simulink model "sscv_braking_ABS_w_vehicle"  (R2024a)
settings: Solver=ode23t  StartTime=0.0  StopTime=1  RelTol=1e-3  AbsTol=1e-3
PreLoadFcn:
  | sscv_braking_ABS_w_vehicle_input
values from neighbouring files (symbols this model uses):
  wheel_rad = 0.3    [sscv_braking_ABS_w_vehicle_input.m]
  wheel_vth = 0.01    [sscv_braking_ABS_w_vehicle_input.m]
undefined symbols (not defined in the file or in its folder): Asphalt, fcdb, HCU, MFormulaCoeff, tpc, vb
libraries: fl_lib x165, SimscapeFluids_lib x24, nesl_utility x21, sdl_lib x9, simulink x3, simulink_extras x1
(part 4 of 6)

== system sscv_braking_ABS_w_vehicle/Road Surface/Road/Select MF Coefficients ==
  Surface : Inport
  Dry Tarmac : Constant  Value=MFormulaCoeff.DryTarmac  SampleTime=0
  Filter MF Coeff LF : Subsystem  mask(First-order lag supporting vector signals){b=0.01, x_initial=MFormulaCoeff.DryTarmac}
      mask prompts: b "Filter time constant"; x_initial "Initial output"
      mask help: Models a lag of the form 1/(b*s+1) where s is the Laplace operator.
  Filter MF Coeff LR : Subsystem  mask(First-order lag supporting vector signals){b=0.01, x_initial=MFormulaCoeff.DryTarmac}
      mask prompts: b "Filter time constant"; x_initial "Initial output"
      mask help: Models a lag of the form 1/(b*s+1) where s is the Laplace operator.
  Filter MF Coeff RF : Subsystem  mask(First-order lag supporting vector signals){b=0.01, x_initial=MFormulaCoeff.DryTarmac}
      mask prompts: b "Filter time constant"; x_initial "Initial output"
      mask help: Models a lag of the form 1/(b*s+1) where s is the Laplace operator.
  Filter MF Coeff RR : Subsystem  mask(First-order lag supporting vector signals){b=0.01, x_initial=MFormulaCoeff.DryTarmac}
      mask prompts: b "Filter time constant"; x_initial "Initial output"
      mask help: Models a lag of the form 1/(b*s+1) where s is the Laplace operator.
  Ice : Constant  Value=MFormulaCoeff.Ice  SampleTime=0
  Select Coeff : Subsystem
  Snow : Constant  Value=MFormulaCoeff.Snow  SampleTime=0
  Wet Tarmac : Constant  Value=MFormulaCoeff.WetTarmac  SampleTime=0
  LF : Outport  VectorParamsAs1DForOutWhenUnconnected=off
  RF : Outport  Port=2  VectorParamsAs1DForOutWhenUnconnected=off
  LR : Outport  Port=3  VectorParamsAs1DForOutWhenUnconnected=off
  RR : Outport  Port=4  VectorParamsAs1DForOutWhenUnconnected=off
  wires:
  Select Coeff/2(RF) -> Filter MF Coeff RF/1(In)
  Select Coeff/1(LF) -> Filter MF Coeff LF/1(In)
  Select Coeff/4(RR) -> Filter MF Coeff RR/1(In)
  Select Coeff/3(LR) -> Filter MF Coeff LR/1(In)
  Surface/1 -> Select Coeff/1(Surface)
  Snow/1 -> Select Coeff/3(Snow)
  Wet Tarmac/1 -> Select Coeff/4(Wet)
  Ice/1 -> Select Coeff/2(Ice)
  Dry Tarmac/1 -> Select Coeff/5(Dry)
  Filter MF Coeff LF/1(Out) -> LF/1
  Filter MF Coeff RF/1(Out) -> RF/1
  Filter MF Coeff LR/1(Out) -> LR/1
  Filter MF Coeff RR/1(Out) -> RR/1

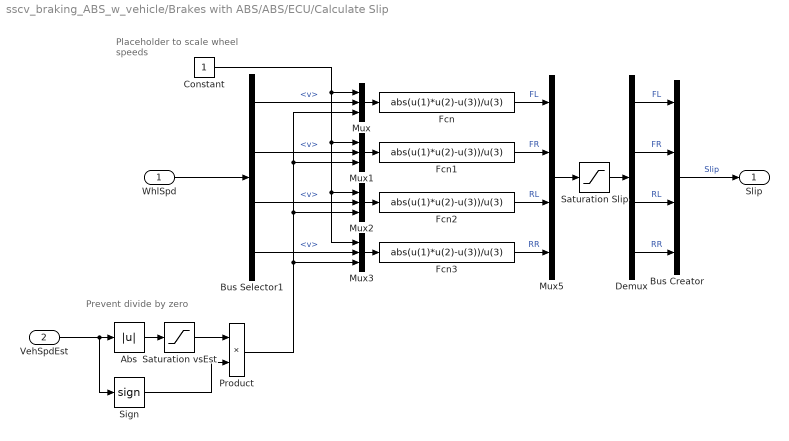
== system sscv_braking_ABS_w_vehicle/Brakes with ABS/ABS/ECU/Calculate Slip ==
  note: Placeholder
      | to scale
      | wheel speeds
  note: Prevent divide by zero
  WhlSpd : Inport
  VehSpdEst : Inport  Port=2
  Abs : Abs  ZeroCross=off  SaturateOnIntegerOverflow=off
  Bus Creator : BusCreator  Inputs=4
  Bus Selector1 : BusSelector  OutputSignals=FL.v,FR.v,RL.v,RR.v
  Constant : Constant
  Demux : Demux
  Fcn{,1..3} (4 alike) : Fcn  Expr=abs(u(1)*u(2)-u(3))/u(3)
  Mux{,1..3} (4 alike) : Mux  Inputs=3
  Mux5 : Mux
  Product : Product
  Saturation Slip : Saturate  UpperLimit=1  LowerLimit=0
  Saturation vsEst : Saturate  UpperLimit=inf  LowerLimit=eps  ZeroCross=off
  Sign : Signum  ZeroCross=off
  Slip : Outport  VectorParamsAs1DForOutWhenUnconnected=off
  wires:
  WhlSpd/1 -> Bus Selector1/1
  Bus Selector1/2 -> Mux1/2  "<v>"
  Bus Selector1/4 -> Mux3/2  "<v>"
  Bus Selector1/1 -> Mux/2  "<v>"
  Bus Selector1/3 -> Mux2/2  "<v>"
  Constant/1 -> Mux1/1, Mux3/1, Mux2/1, Mux/1
  VehSpdEst/1 -> Sign/1, Abs/1
  Demux/1 -> Bus Creator/1  "FL"
  Demux/2 -> Bus Creator/2  "FR"
  Demux/3 -> Bus Creator/3  "RL"
  Demux/4 -> Bus Creator/4  "RR"
  Bus Creator/1 -> Slip/1  "Slip"
  Product/1 -> Mux3/3, Mux2/3, Mux1/3, Mux/3
  Abs/1 -> Saturation vsEst/1
  Saturation vsEst/1 -> Product/1
  Sign/1 -> Product/2
  Mux/1 -> Fcn/1
  Mux1/1 -> Fcn1/1
  Mux2/1 -> Fcn2/1
  Mux3/1 -> Fcn3/1
  Mux5/1 -> Saturation Slip/1
  Saturation Slip/1 -> Demux/1
  Fcn/1 -> Mux5/1  "FL"
  Fcn1/1 -> Mux5/2  "FR"
  Fcn2/1 -> Mux5/3  "RL"
  Fcn3/1 -> Mux5/4  "RR"

== system sscv_braking_ABS_w_vehicle/Brakes with ABS/ABS/ECU/Valve Control FL ==
  Slip : Inport
  vSpdEst : Inport  Port=2
  Code to Valves : Subsystem
  Demux : Demux  Outputs=2
  Logic : Stateflow chart  TreatAsAtomicUnit=on
  Mux : Mux  Inputs=2
  Product : Product
  Subsystem : Subsystem
  Subsystem1 : Subsystem
  Valve : Outport  VectorParamsAs1DForOutWhenUnconnected=off
  wires:
  Subsystem1/1(vSig) -> Mux/2
  Subsystem/1(vSig) -> Mux/1
  Mux/1 -> Valve/1
  Demux/2 -> Subsystem1/1(OnT)
  Demux/1 -> Subsystem/1(OnT)
  Product/1 -> Demux/1
  vSpdEst/1 -> Logic/2(vSpdEst)
  Code to Valves/1(V) -> Product/1
  Slip/1 -> Logic/1(Slip)
  Logic/2(Mod_Dur) -> Product/2
  Logic/1(Mod_State) -> Code to Valves/1(C)

== system sscv_braking_ABS_w_vehicle/Brakes with ABS/ABS/ECU/Valve Control FR ==
  Slip : Inport
  vSpdEst : Inport  Port=2
  Code to Valves : Subsystem
  Demux : Demux  Outputs=2
  Logic : Stateflow chart  TreatAsAtomicUnit=on
  Mux : Mux  Inputs=2
  Product : Product
  Subsystem : Subsystem
  Subsystem1 : Subsystem
  Valve : Outport  VectorParamsAs1DForOutWhenUnconnected=off
  wires:
  Subsystem1/1(vSig) -> Mux/2
  Subsystem/1(vSig) -> Mux/1
  Mux/1 -> Valve/1
  Demux/2 -> Subsystem1/1(OnT)
  Demux/1 -> Subsystem/1(OnT)
  Product/1 -> Demux/1
  vSpdEst/1 -> Logic/2(vSpdEst)
  Code to Valves/1(V) -> Product/1
  Slip/1 -> Logic/1(Slip)
  Logic/2(Mod_Dur) -> Product/2
  Logic/1(Mod_State) -> Code to Valves/1(C)

== system sscv_braking_ABS_w_vehicle/Brakes with ABS/ABS/ECU/Valve Control RL ==
  Slip : Inport
  vSpdEst : Inport  Port=2
  Code to Valves : Subsystem
  Demux : Demux  Outputs=2
  Logic : Stateflow chart  TreatAsAtomicUnit=on
  Mux : Mux  Inputs=2
  Product : Product
  Subsystem : Subsystem
  Subsystem1 : Subsystem
  Valve : Outport  VectorParamsAs1DForOutWhenUnconnected=off
  wires:
  Subsystem1/1(vSig) -> Mux/2
  Subsystem/1(vSig) -> Mux/1
  Mux/1 -> Valve/1
  Demux/2 -> Subsystem1/1(OnT)
  Demux/1 -> Subsystem/1(OnT)
  Product/1 -> Demux/1
  vSpdEst/1 -> Logic/2(vSpdEst)
  Code to Valves/1(V) -> Product/1
  Slip/1 -> Logic/1(Slip)
  Logic/2(Mod_Dur) -> Product/2
  Logic/1(Mod_State) -> Code to Valves/1(C)

== system sscv_braking_ABS_w_vehicle/Brakes with ABS/ABS/ECU/Valve Control RR ==
  Slip : Inport
  vSpdEst : Inport  Port=2
  Code to Valves : Subsystem
  Demux : Demux  Outputs=2
  Logic : Stateflow chart  TreatAsAtomicUnit=on
  Mux : Mux  Inputs=2
  Product : Product
  Subsystem : Subsystem
  Subsystem1 : Subsystem
  Valve : Outport  VectorParamsAs1DForOutWhenUnconnected=off
  wires:
  Subsystem1/1(vSig) -> Mux/2
  Subsystem/1(vSig) -> Mux/1
  Mux/1 -> Valve/1
  Demux/2 -> Subsystem1/1(OnT)
  Demux/1 -> Subsystem/1(OnT)
  Product/1 -> Demux/1
  vSpdEst/1 -> Logic/2(vSpdEst)
  Code to Valves/1(V) -> Product/1
  Slip/1 -> Logic/1(Slip)
  Logic/2(Mod_Dur) -> Product/2
  Logic/1(Mod_State) -> Code to Valves/1(C)

== system sscv_braking_ABS_w_vehicle/Brakes with ABS/ABS/ECU/Vehicle Speed ==
  note: Estimates wheel speed using only wheel speed sensors and longitudinal accelerometer.
  note: Longitudinal
      | Accelerometer
  Sensors : Inport
  Accelerometer : simulink_extras/Additional Linear/Transfer Fcn (with initial states)  N=[1 0]  D="[0.01  1]"  X0=0
  Bus Selector : BusSelector  OutputSignals=v
  Bus Selector1 : BusSelector  OutputSignals=FL.v,FR.v,RL.v,RR.v
  Dynamic Rate Limiter : Subsystem
  Max : MinMax  Function=max  Inputs=4
  Rate Limit high : Constant  Value=8
  Saturation : Saturate  UpperLimit=0  LowerLimit=-inf
  ZOH rate limit low : ZeroOrderHold  SampleTime=1e-2
  ZOH vel : ZeroOrderHold  SampleTime=1e-2
  vSpdEst : Outport  VectorParamsAs1DForOutWhenUnconnected=off
  wires:
  Sensors/1 -> Bus Selector/1, Bus Selector1/1
  Bus Selector/1 -> Accelerometer/1  "<v>"
  Bus Selector1/1 -> Max/1  "<v>"
  Bus Selector1/2 -> Max/2  "<v>"
  Bus Selector1/3 -> Max/3  "<v>"
  Bus Selector1/4 -> Max/4  "<v>"
  Max/1 -> ZOH vel/1  "Max Wheel Spd"
  ZOH vel/1 -> Dynamic Rate Limiter/2(u)
  ZOH rate limit low/1 -> Dynamic Rate Limiter/3(lo)
  Rate Limit high/1 -> Dynamic Rate Limiter/1(up)
  Dynamic Rate Limiter/1(Y) -> vSpdEst/1  "vSpdEst"
  Accelerometer/1 -> Saturation/1
  Saturation/1 -> ZOH rate limit low/1

== system sscv_braking_ABS_w_vehicle/Brakes with ABS/ABS/HCU/Actuator Dynamics FL ==
  In : Inport
  Gain : Gain  Gain=1./b
  Integrator : Integrator  InitialCondition=x_initial.*b
  Sum : Sum  Inputs=|+-  InputSameDT=on  SaturateOnIntegerOverflow=on  OutDataTypeStr=Inherit: Same as first input
  Out : Outport  VectorParamsAs1DForOutWhenUnconnected=off
  wires:
  Sum/1 -> Integrator/1
  In/1 -> Sum/1
  Integrator/1 -> Gain/1
  Gain/1 -> Sum/2, Out/1

== system sscv_braking_ABS_w_vehicle/Brakes with ABS/ABS/HCU/Actuator Dynamics FR ==
  In : Inport
  Gain : Gain  Gain=1./b
  Integrator : Integrator  InitialCondition=x_initial.*b
  Sum : Sum  Inputs=|+-  InputSameDT=on  SaturateOnIntegerOverflow=on  OutDataTypeStr=Inherit: Same as first input
  Out : Outport  VectorParamsAs1DForOutWhenUnconnected=off
  wires:
  Gain/1 -> Out/1, Sum/2
  Integrator/1 -> Gain/1
  In/1 -> Sum/1
  Sum/1 -> Integrator/1

== system sscv_braking_ABS_w_vehicle/Brakes with ABS/ABS/HCU/Actuator Dynamics RL ==
  In : Inport
  Gain : Gain  Gain=1./b
  Integrator : Integrator  InitialCondition=x_initial.*b
  Sum : Sum  Inputs=|+-  InputSameDT=on  SaturateOnIntegerOverflow=on  OutDataTypeStr=Inherit: Same as first input
  Out : Outport  VectorParamsAs1DForOutWhenUnconnected=off
  wires:
  Gain/1 -> Out/1, Sum/2
  Integrator/1 -> Gain/1
  In/1 -> Sum/1
  Sum/1 -> Integrator/1

== system sscv_braking_ABS_w_vehicle/Brakes with ABS/ABS/HCU/Actuator Dynamics RR ==
  In : Inport
  Gain : Gain  Gain=1./b
  Integrator : Integrator  InitialCondition=x_initial.*b
  Sum : Sum  Inputs=|+-  InputSameDT=on  SaturateOnIntegerOverflow=on  OutDataTypeStr=Inherit: Same as first input
  Out : Outport  VectorParamsAs1DForOutWhenUnconnected=off
  wires:
  Gain/1 -> Out/1, Sum/2
  Integrator/1 -> Gain/1
  In/1 -> Sum/1
  Sum/1 -> Integrator/1

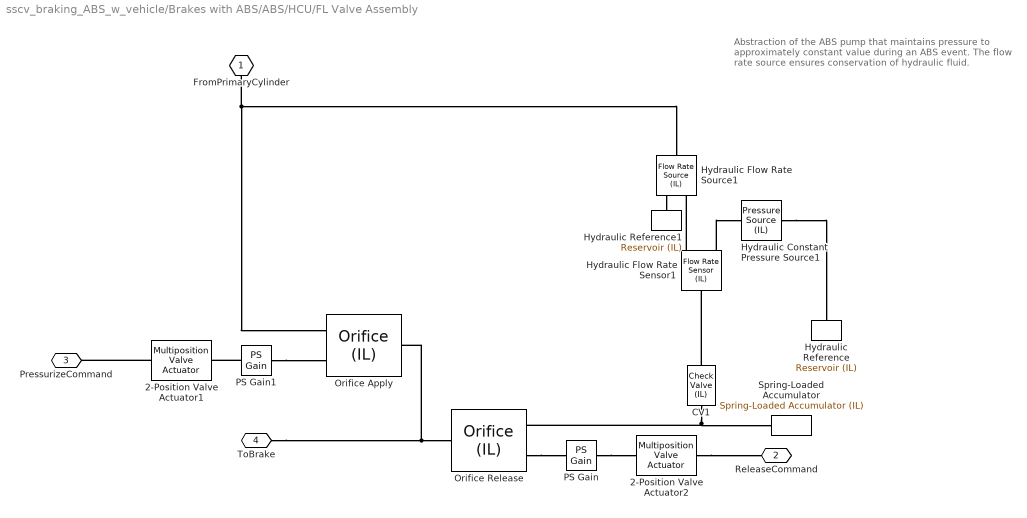
== system sscv_braking_ABS_w_vehicle/Brakes with ABS/ABS/HCU/FL Valve Assembly ==
  note: Abstraction of the ABS pump
      | that maintains pressure to
      | approximately constant value
      | during an ABS event. The
      | flow rate source ensures
      | conservation of hydraulic fluid.
  2-Position Valve Actuator1 : SimscapeFluids_lib/Valve Actuators/Multiposition Valve Actuator  positions=fluids.valve_actuators.enum.actuator_num_positions.two  stroke=HCU.PushPinS m  t_on=HCU.SwitchOnT s  t_off=HCU.SwitchOffT s  act_signal=HCU.NomSigV  init_position_2=0  init_position_3=fluids.valve_actuators.enum.actuator_three_pos_ic.neutral  act_orientation=1  local_time_specify=off  local_time_priority=None  local_time=0 s  local_time_nominal_specify=off  local_time_nominal_value=1  local_time_nominal_unit=s
      settings: InternalSimscapePortConfiguration="{\"Bottom\":[],\"Left\":[{\"id\":\"A\",\"label\":\"A\",\"type\":\"input\"}],\"Right\":[{\"id\":\"S\",\"label\":\"S\",\"type\":\"output\"}],\"Top\":[]}"
  2-Position Valve Actuator2 : SimscapeFluids_lib/Valve Actuators/Multiposition Valve Actuator  positions=fluids.valve_actuators.enum.actuator_num_positions.two  stroke=HCU.PushPinS m  t_on=HCU.SwitchOnT s  t_off=HCU.SwitchOffT s  act_signal=HCU.NomSigV  init_position_2=0  init_position_3=fluids.valve_actuators.enum.actuator_three_pos_ic.neutral  act_orientation=1  local_time_specify=off  local_time_priority=None  local_time=0 s  local_time_nominal_specify=off  local_time_nominal_value=1  local_time_nominal_unit=s
      settings: InternalSimscapePortConfiguration="{\"Bottom\":[],\"Left\":[{\"id\":\"A\",\"label\":\"A\",\"type\":\"input\"}],\"Right\":[{\"id\":\"S\",\"label\":\"S\",\"type\":\"output\"}],\"Top\":[]}"
  CV1 : SimscapeFluids_lib/Isothermal Liquid/Valves & Orifices/Directional Control Valves/Check Valve (IL)  opening_spec=fluids.isothermal_liquid.valves_orifices.enum.PressureOpeningSpec.Linear  pressure_control_spec=fluids.isothermal_liquid.valves_orifices.enum.pressure_control_spec.dp  p_crack_differential=HCU.cv1CrackP Pa  p_crack_gauge=0.1 MPa  press_max_differential=HCU.cv1MaxOpP Pa  press_max_gauge=0.2 MPa  area_max=HCU.cv1Amax m^2  area_leak=1e-8 m^2  p_diff_TLU=[0.01 : 0.01 : 0.1] MPa  valve_area_TLU=[1e-10, 1e-05, 2e-05, 3e-05, 4e-05, 5e-05, 6e-05, 7.5e-05, 8.5e-05, .0001] m^2  vol_flow_TLU=[.000358, .045, .11, .191, .284, .39, .505, .63, .764, .905] .* 1e-3 m^3/s  area=inf m^2  Cd=0.7  Re_c=150  smoothing_factor=0  pressure_recovery=simscape.enum.onoff.off  opening_dynamics=0  tau=0.1 s  enable_faults=simscape.enum.onoff.off  fault_action=fluids.enum.FaultOpening.Closed
      settings: InternalSimscapePortConfiguration="{\"Bottom\":[],\"Left\":[{\"id\":\"A\",\"label\":\"A\",\"type\":\"foundation.isothermal_liquid.isothermal_liquid\"}],\"Right\":[{\"id\":\"B\",\"label\":\"B\",\"type\":\"foundation.isothermal_liquid.isothermal_liquid\"}],\"Top\":[]}"
  Hydraulic Constant Pressure Source1 : fl_lib/Isothermal Liquid/Sources/Pressure Source (IL)  source_type=1  pressure_differential=1 atm
      settings: InternalSimscapePortConfiguration="{\"Bottom\":[],\"Left\":[{\"id\":\"A\",\"label\":\"A\",\"type\":\"foundation.isothermal_liquid.isothermal_liquid\"}],\"Right\":[{\"id\":\"B\",\"label\":\"B\",\"type\":\"foundation.isothermal_liquid.isothermal_liquid\"}],\"Top\":[]}"
  Hydraulic Flow Rate Sensor1 : fl_lib/Isothermal Liquid/Sensors/Flow Rate Sensor (IL)  sensor_type=3
      settings: InternalSimscapePortConfiguration="{\"Bottom\":[],\"Left\":[{\"id\":\"A\",\"label\":\"A\",\"type\":\"foundation.isothermal_liquid.isothermal_liquid\"}],\"Right\":[{\"id\":\"B\",\"label\":\"B\",\"type\":\"foundation.isothermal_liquid.isothermal_liquid\"},{\"id\":\"M\",\"label\":\"M\",\"type\":\"output\"},{\"id\":\"V\",\"label\":\"V\",\"type\":\"output\"}],\"Top\":[]}"
  Hydraulic Flow Rate Source1 : fl_lib/Isothermal Liquid/Sources/Flow Rate Source (IL)  source_type=foundation.enum.constant_controlled.controlled  flow_type=2  mass_flow=0 kg/s  volumetric_flow=0 m^3/s
      settings: InternalSimscapePortConfiguration="{\"Bottom\":[],\"Left\":[{\"id\":\"A\",\"label\":\"A\",\"type\":\"foundation.isothermal_liquid.isothermal_liquid\"},{\"id\":\"V\",\"label\":\"V\",\"type\":\"input\"}],\"Right\":[{\"id\":\"B\",\"label\":\"B\",\"type\":\"foundation.isothermal_liquid.isothermal_liquid\"}],\"Top\":[]}"
  Hydraulic Reference : fl_lib/Isothermal Liquid/Elements/Reservoir (IL)  reservoir_type=foundation.enum.constant_controlled.constant  pressure_spec=foundation.enum.pressure_spec.atmospheric  reservoir_pressure=0.101325 MPa
  Hydraulic Reference1 : fl_lib/Isothermal Liquid/Elements/Reservoir (IL)  reservoir_type=foundation.enum.constant_controlled.constant  pressure_spec=foundation.enum.pressure_spec.atmospheric  reservoir_pressure=0.101325 MPa
  Orifice Apply : SimscapeFluids_lib/Isothermal Liquid/Valves & Orifices/Orifices/Orifice (IL)  orifice_type=foundation.enum.constant_variable.variable  constant_orifice_spec=fluids.isothermal_liquid.valves_orifices.orifices.enum.constant_orifice_spec.area  variable_orifice_spec=1  orifice_area_constant=1e-3 m^2  p_diff_TLU_constant=[-4, -3, -2, -1, -.5, 0, .5, 1, 2, 3, 4] MPa  vol_flow_TLU_constant=[-2.44, -2.12, -1.68, -1.22, -.84, 0, .85, 1.21, 1.7, 2.09, 2.41] .* 1e-3 m^3/s  S_min=HCU.valve_x0 m  del_S=HCU.valve_maxO m  open_orientation=1  area_max=HCU.valve_maxA m^2  area_leak=HCU.valve_leak m^2  S_TLU=[-.002, 0, .002, .005, .015] - (HCU.valve_x0) m  orifice_area_TLU=[1e-09, 2.0352e-07, 4.0736e-05, .00011438, .00034356] m^2  area=inf m^2  Cd=0.7  Re_c=150  smoothing_factor=0  pressure_recovery=simscape.enum.onoff.off  S_vol_flow_TLU=[-.002, 0, .002, .005, .015] - (HCU.valve_x0) m  p_diff_TLU=[-10000000, -5000000, -2000000, 2000000, 5000000, 10000000] Pa  vol_flow_TLU=[-1e-07, -7.0711e-08, -4.4721e-08, 4.4721e-08, 7.0711e-08, 1e-07; -2.0352e-05, -1.4391e-05, -9.1017e-06, 9.1017e-06, 1.4391e-05, 2.0352e-05; -.0040736, -.0028805, -.0018218, .0018218, .0028805, .0040736; -.011438, -.0080879, -.0051152, .0051152, .0080879, .011438; -.034356, -.024293, -.015364, .015364, .024293, .034356] m^3/s  enable_faults=simscape.enum.onoff.off  fault_action=fluids.enum.FaultOpening.Closed
      settings: InternalSimscapePortConfiguration="{\"Bottom\":[],\"Left\":[{\"id\":\"A\",\"label\":\"A\",\"type\":\"foundation.isothermal_liquid.isothermal_liquid\"},{\"id\":\"S\",\"label\":\"S\",\"type\":\"input\"}],\"Right\":[{\"id\":\"B\",\"label\":\"B\",\"type\":\"foundation.isothermal_liquid.isothermal_liquid\"}],\"Top\":[]}"
  Orifice Release : SimscapeFluids_lib/Isothermal Liquid/Valves & Orifices/Orifices/Orifice (IL)  orifice_type=foundation.enum.constant_variable.variable  constant_orifice_spec=fluids.isothermal_liquid.valves_orifices.orifices.enum.constant_orifice_spec.area  variable_orifice_spec=1  orifice_area_constant=1e-3 m^2  p_diff_TLU_constant=[-4, -3, -2, -1, -.5, 0, .5, 1, 2, 3, 4] MPa  vol_flow_TLU_constant=[-2.44, -2.12, -1.68, -1.22, -.84, 0, .85, 1.21, 1.7, 2.09, 2.41] .* 1e-3 m^3/s  S_min=HCU.valve_x0 m  del_S=HCU.valve_maxO m  open_orientation=1  area_max=HCU.valve_maxA m^2  area_leak=HCU.valve_leak m^2  S_TLU=[-.002, 0, .002, .005, .015] - (HCU.valve_x0) m  orifice_area_TLU=[1e-09, 2.0352e-07, 4.0736e-05, .00011438, .00034356] m^2  area=inf m^2  Cd=0.7  Re_c=150  smoothing_factor=0  pressure_recovery=simscape.enum.onoff.off  S_vol_flow_TLU=[-.002, 0, .002, .005, .015] - (HCU.valve_x0) m  p_diff_TLU=[-10000000, -5000000, -2000000, 2000000, 5000000, 10000000] Pa  vol_flow_TLU=[-1e-07, -7.0711e-08, -4.4721e-08, 4.4721e-08, 7.0711e-08, 1e-07; -2.0352e-05, -1.4391e-05, -9.1017e-06, 9.1017e-06, 1.4391e-05, 2.0352e-05; -.0040736, -.0028805, -.0018218, .0018218, .0028805, .0040736; -.011438, -.0080879, -.0051152, .0051152, .0080879, .011438; -.034356, -.024293, -.015364, .015364, .024293, .034356] m^3/s  enable_faults=simscape.enum.onoff.off  fault_action=fluids.enum.FaultOpening.Closed
      settings: InternalSimscapePortConfiguration="{\"Bottom\":[],\"Left\":[{\"id\":\"A\",\"label\":\"A\",\"type\":\"foundation.isothermal_liquid.isothermal_liquid\"},{\"id\":\"S\",\"label\":\"S\",\"type\":\"input\"}],\"Right\":[{\"id\":\"B\",\"label\":\"B\",\"type\":\"foundation.isothermal_liquid.isothermal_liquid\"}],\"Top\":[]}"
  PS Gain : fl_lib/Physical Signals/Functions/PS Gain  gain=HCU.valve_maxO
  PS Gain1 : fl_lib/Physical Signals/Functions/PS Gain  gain=HCU.valve_maxO
  Spring-Loaded Accumulator : SimscapeFluids_lib/Isothermal Liquid/Tanks & Accumulators/Spring-Loaded Accumulator (IL)  capacity=HCU.FluidChamC cm^3  p_preload="HCU.PrelP  bar"  p_max="HCU.FullCapP  bar"  stiff_coeff=HCU.hss Pa/m^3  dynamic_compressibility=simscape.enum.onoff.off  liquid_volume_specify=on  liquid_volume_priority=High  liquid_volume=0 m^3  liquid_volume_nominal_specify=off  liquid_volume_nominal_value=1  liquid_volume_nominal_unit=m^3  liquid_mass_specify=off  liquid_mass_priority=None  liquid_mass=5 kg  liquid_mass_nominal_specify=off  liquid_mass_nominal_value=1  liquid_mass_nominal_unit=kg  p_I_specify=on  p_I_priority=None  p_I=1.01325e5 Pa  p_I_nominal_specify=off  p_I_nominal_value=1  p_I_nominal_unit=Pa
      settings: InternalSimscapePortConfiguration="{\"Bottom\":[],\"Left\":[],\"Right\":[{\"id\":\"A\",\"label\":\"A\",\"type\":\"foundation.isothermal_liquid.isothermal_liquid\"}],\"Top\":[]}"
  FromPrimaryCylinder : PMIOPort  Side=Left
  ReleaseCommand : PMIOPort  Port=2  Side=Left
  PressurizeCommand : PMIOPort  Port=3  Side=Left
  ToBrake : PMIOPort  Port=4  Side=Right
  connections:
  2-Position Valve Actuator2/LConn1 -- ReleaseCommand/RConn1
  PS Gain/LConn1 -- 2-Position Valve Actuator2/RConn1
  2-Position Valve Actuator1/LConn1 -- PressurizeCommand/RConn1
  PS Gain1/LConn1 -- 2-Position Valve Actuator1/RConn1
  Hydraulic Constant Pressure Source1/LConn1 -- Hydraulic Reference/LConn1
  Hydraulic Flow Rate Source1/LConn1 -- Hydraulic Reference1/LConn1
  Hydraulic Flow Rate Sensor1/RConn3 -- Hydraulic Flow Rate Source1/LConn2
  Orifice Release/LConn2 -- PS Gain/RConn1
  PS Gain1/RConn1 -- Orifice Apply/LConn2
  CV1/LConn1 -- Spring-Loaded Accumulator/RConn1 -- Orifice Release/LConn1
  ToBrake/RConn1 -- Orifice Release/RConn1 -- Orifice Apply/RConn1
  FromPrimaryCylinder/RConn1 -- Orifice Apply/LConn1 -- Hydraulic Flow Rate Source1/RConn1
  Hydraulic Flow Rate Sensor1/RConn1 -- Hydraulic Constant Pressure Source1/RConn1
  CV1/RConn1 -- Hydraulic Flow Rate Sensor1/LConn1

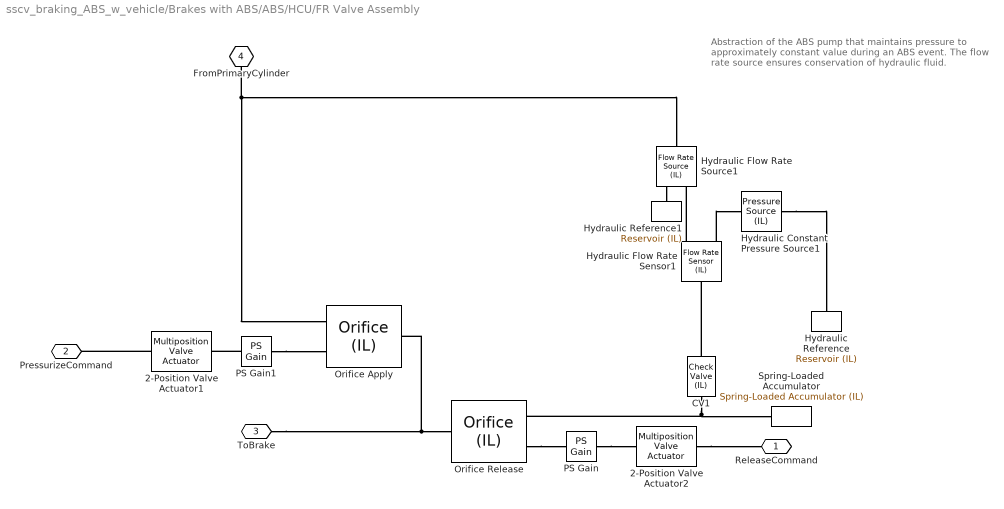
== system sscv_braking_ABS_w_vehicle/Brakes with ABS/ABS/HCU/FR Valve Assembly ==
  note: Abstraction of the ABS pump
      | that maintains pressure to
      | approximately constant value
      | during an ABS event. The
      | flow rate source ensures
      | conservation of hydraulic fluid.
  2-Position Valve Actuator1 : SimscapeFluids_lib/Valve Actuators/Multiposition Valve Actuator  positions=fluids.valve_actuators.enum.actuator_num_positions.two  stroke=HCU.PushPinS m  t_on=HCU.SwitchOnT s  t_off=HCU.SwitchOffT s  act_signal=HCU.NomSigV  init_position_2=0  init_position_3=fluids.valve_actuators.enum.actuator_three_pos_ic.neutral  act_orientation=1  local_time_specify=off  local_time_priority=None  local_time=0 s  local_time_nominal_specify=off  local_time_nominal_value=1  local_time_nominal_unit=s
      settings: InternalSimscapePortConfiguration="{\"Bottom\":[],\"Left\":[{\"id\":\"A\",\"label\":\"A\",\"type\":\"input\"}],\"Right\":[{\"id\":\"S\",\"label\":\"S\",\"type\":\"output\"}],\"Top\":[]}"
  2-Position Valve Actuator2 : SimscapeFluids_lib/Valve Actuators/Multiposition Valve Actuator  positions=fluids.valve_actuators.enum.actuator_num_positions.two  stroke=HCU.PushPinS m  t_on=HCU.SwitchOnT s  t_off=HCU.SwitchOffT s  act_signal=HCU.NomSigV  init_position_2=0  init_position_3=fluids.valve_actuators.enum.actuator_three_pos_ic.neutral  act_orientation=1  local_time_specify=off  local_time_priority=None  local_time=0 s  local_time_nominal_specify=off  local_time_nominal_value=1  local_time_nominal_unit=s
      settings: InternalSimscapePortConfiguration="{\"Bottom\":[],\"Left\":[{\"id\":\"A\",\"label\":\"A\",\"type\":\"input\"}],\"Right\":[{\"id\":\"S\",\"label\":\"S\",\"type\":\"output\"}],\"Top\":[]}"
  CV1 : SimscapeFluids_lib/Isothermal Liquid/Valves & Orifices/Directional Control Valves/Check Valve (IL)  opening_spec=fluids.isothermal_liquid.valves_orifices.enum.PressureOpeningSpec.Linear  pressure_control_spec=fluids.isothermal_liquid.valves_orifices.enum.pressure_control_spec.dp  p_crack_differential=HCU.cv1CrackP Pa  p_crack_gauge=0.1 MPa  press_max_differential=HCU.cv1MaxOpP Pa  press_max_gauge=0.2 MPa  area_max=HCU.cv1Amax m^2  area_leak=1e-8 m^2  p_diff_TLU=[0.01 : 0.01 : 0.1] MPa  valve_area_TLU=[1e-10, 1e-05, 2e-05, 3e-05, 4e-05, 5e-05, 6e-05, 7.5e-05, 8.5e-05, .0001] m^2  vol_flow_TLU=[.000358, .045, .11, .191, .284, .39, .505, .63, .764, .905] .* 1e-3 m^3/s  area=inf m^2  Cd=0.7  Re_c=150  smoothing_factor=0  pressure_recovery=simscape.enum.onoff.off  opening_dynamics=0  tau=0.1 s  enable_faults=simscape.enum.onoff.off  fault_action=fluids.enum.FaultOpening.Closed
      settings: InternalSimscapePortConfiguration="{\"Bottom\":[],\"Left\":[{\"id\":\"A\",\"label\":\"A\",\"type\":\"foundation.isothermal_liquid.isothermal_liquid\"}],\"Right\":[{\"id\":\"B\",\"label\":\"B\",\"type\":\"foundation.isothermal_liquid.isothermal_liquid\"}],\"Top\":[]}"
  Hydraulic Constant Pressure Source1 : fl_lib/Isothermal Liquid/Sources/Pressure Source (IL)  source_type=1  pressure_differential=1 atm
      settings: InternalSimscapePortConfiguration="{\"Bottom\":[],\"Left\":[{\"id\":\"A\",\"label\":\"A\",\"type\":\"foundation.isothermal_liquid.isothermal_liquid\"}],\"Right\":[{\"id\":\"B\",\"label\":\"B\",\"type\":\"foundation.isothermal_liquid.isothermal_liquid\"}],\"Top\":[]}"
  Hydraulic Flow Rate Sensor1 : fl_lib/Isothermal Liquid/Sensors/Flow Rate Sensor (IL)  sensor_type=3
      settings: InternalSimscapePortConfiguration="{\"Bottom\":[],\"Left\":[{\"id\":\"A\",\"label\":\"A\",\"type\":\"foundation.isothermal_liquid.isothermal_liquid\"}],\"Right\":[{\"id\":\"B\",\"label\":\"B\",\"type\":\"foundation.isothermal_liquid.isothermal_liquid\"},{\"id\":\"M\",\"label\":\"M\",\"type\":\"output\"},{\"id\":\"V\",\"label\":\"V\",\"type\":\"output\"}],\"Top\":[]}"
  Hydraulic Flow Rate Source1 : fl_lib/Isothermal Liquid/Sources/Flow Rate Source (IL)  source_type=foundation.enum.constant_controlled.controlled  flow_type=2  mass_flow=0 kg/s  volumetric_flow=0 m^3/s
      settings: InternalSimscapePortConfiguration="{\"Bottom\":[],\"Left\":[{\"id\":\"A\",\"label\":\"A\",\"type\":\"foundation.isothermal_liquid.isothermal_liquid\"},{\"id\":\"V\",\"label\":\"V\",\"type\":\"input\"}],\"Right\":[{\"id\":\"B\",\"label\":\"B\",\"type\":\"foundation.isothermal_liquid.isothermal_liquid\"}],\"Top\":[]}"
  Hydraulic Reference : fl_lib/Isothermal Liquid/Elements/Reservoir (IL)  reservoir_type=foundation.enum.constant_controlled.constant  pressure_spec=foundation.enum.pressure_spec.atmospheric  reservoir_pressure=0.101325 MPa
  Hydraulic Reference1 : fl_lib/Isothermal Liquid/Elements/Reservoir (IL)  reservoir_type=foundation.enum.constant_controlled.constant  pressure_spec=foundation.enum.pressure_spec.atmospheric  reservoir_pressure=0.101325 MPa
  Orifice Apply : SimscapeFluids_lib/Isothermal Liquid/Valves & Orifices/Orifices/Orifice (IL)  orifice_type=foundation.enum.constant_variable.variable  constant_orifice_spec=fluids.isothermal_liquid.valves_orifices.orifices.enum.constant_orifice_spec.area  variable_orifice_spec=1  orifice_area_constant=1e-3 m^2  p_diff_TLU_constant=[-4, -3, -2, -1, -.5, 0, .5, 1, 2, 3, 4] MPa  vol_flow_TLU_constant=[-2.44, -2.12, -1.68, -1.22, -.84, 0, .85, 1.21, 1.7, 2.09, 2.41] .* 1e-3 m^3/s  S_min=HCU.valve_x0 m  del_S=HCU.valve_maxO m  open_orientation=1  area_max=HCU.valve_maxA m^2  area_leak=HCU.valve_leak m^2  S_TLU=[-.002, 0, .002, .005, .015] - (HCU.valve_x0) m  orifice_area_TLU=[1e-09, 2.0352e-07, 4.0736e-05, .00011438, .00034356] m^2  area=inf m^2  Cd=0.7  Re_c=150  smoothing_factor=0  pressure_recovery=simscape.enum.onoff.off  S_vol_flow_TLU=[-.002, 0, .002, .005, .015] - (HCU.valve_x0) m  p_diff_TLU=[-10000000, -5000000, -2000000, 2000000, 5000000, 10000000] Pa  vol_flow_TLU=[-1e-07, -7.0711e-08, -4.4721e-08, 4.4721e-08, 7.0711e-08, 1e-07; -2.0352e-05, -1.4391e-05, -9.1017e-06, 9.1017e-06, 1.4391e-05, 2.0352e-05; -.0040736, -.0028805, -.0018218, .0018218, .0028805, .0040736; -.011438, -.0080879, -.0051152, .0051152, .0080879, .011438; -.034356, -.024293, -.015364, .015364, .024293, .034356] m^3/s  enable_faults=simscape.enum.onoff.off  fault_action=fluids.enum.FaultOpening.Closed
      settings: InternalSimscapePortConfiguration="{\"Bottom\":[],\"Left\":[{\"id\":\"A\",\"label\":\"A\",\"type\":\"foundation.isothermal_liquid.isothermal_liquid\"},{\"id\":\"S\",\"label\":\"S\",\"type\":\"input\"}],\"Right\":[{\"id\":\"B\",\"label\":\"B\",\"type\":\"foundation.isothermal_liquid.isothermal_liquid\"}],\"Top\":[]}"
  Orifice Release : SimscapeFluids_lib/Isothermal Liquid/Valves & Orifices/Orifices/Orifice (IL)  orifice_type=foundation.enum.constant_variable.variable  constant_orifice_spec=fluids.isothermal_liquid.valves_orifices.orifices.enum.constant_orifice_spec.area  variable_orifice_spec=1  orifice_area_constant=1e-3 m^2  p_diff_TLU_constant=[-4, -3, -2, -1, -.5, 0, .5, 1, 2, 3, 4] MPa  vol_flow_TLU_constant=[-2.44, -2.12, -1.68, -1.22, -.84, 0, .85, 1.21, 1.7, 2.09, 2.41] .* 1e-3 m^3/s  S_min=HCU.valve_x0 m  del_S=HCU.valve_maxO m  open_orientation=1  area_max=HCU.valve_maxA m^2  area_leak=HCU.valve_leak m^2  S_TLU=[-.002, 0, .002, .005, .015] - (HCU.valve_x0) m  orifice_area_TLU=[1e-09, 2.0352e-07, 4.0736e-05, .00011438, .00034356] m^2  area=inf m^2  Cd=0.7  Re_c=150  smoothing_factor=0  pressure_recovery=simscape.enum.onoff.off  S_vol_flow_TLU=[-.002, 0, .002, .005, .015] - (HCU.valve_x0) m  p_diff_TLU=[-10000000, -5000000, -2000000, 2000000, 5000000, 10000000] Pa  vol_flow_TLU=[-1e-07, -7.0711e-08, -4.4721e-08, 4.4721e-08, 7.0711e-08, 1e-07; -2.0352e-05, -1.4391e-05, -9.1017e-06, 9.1017e-06, 1.4391e-05, 2.0352e-05; -.0040736, -.0028805, -.0018218, .0018218, .0028805, .0040736; -.011438, -.0080879, -.0051152, .0051152, .0080879, .011438; -.034356, -.024293, -.015364, .015364, .024293, .034356] m^3/s  enable_faults=simscape.enum.onoff.off  fault_action=fluids.enum.FaultOpening.Closed
      settings: InternalSimscapePortConfiguration="{\"Bottom\":[],\"Left\":[{\"id\":\"A\",\"label\":\"A\",\"type\":\"foundation.isothermal_liquid.isothermal_liquid\"},{\"id\":\"S\",\"label\":\"S\",\"type\":\"input\"}],\"Right\":[{\"id\":\"B\",\"label\":\"B\",\"type\":\"foundation.isothermal_liquid.isothermal_liquid\"}],\"Top\":[]}"
  PS Gain : fl_lib/Physical Signals/Functions/PS Gain  gain=HCU.valve_maxO
  PS Gain1 : fl_lib/Physical Signals/Functions/PS Gain  gain=HCU.valve_maxO
  Spring-Loaded Accumulator : SimscapeFluids_lib/Isothermal Liquid/Tanks & Accumulators/Spring-Loaded Accumulator (IL)  capacity=HCU.FluidChamC cm^3  p_preload="HCU.PrelP  bar"  p_max="HCU.FullCapP  bar"  stiff_coeff=HCU.hss Pa/m^3  dynamic_compressibility=simscape.enum.onoff.off  liquid_volume_specify=on  liquid_volume_priority=High  liquid_volume=0 m^3  liquid_volume_nominal_specify=off  liquid_volume_nominal_value=1  liquid_volume_nominal_unit=m^3  liquid_mass_specify=off  liquid_mass_priority=None  liquid_mass=5 kg  liquid_mass_nominal_specify=off  liquid_mass_nominal_value=1  liquid_mass_nominal_unit=kg  p_I_specify=on  p_I_priority=None  p_I=1.01325e5 Pa  p_I_nominal_specify=off  p_I_nominal_value=1  p_I_nominal_unit=Pa
      settings: InternalSimscapePortConfiguration="{\"Bottom\":[],\"Left\":[],\"Right\":[{\"id\":\"A\",\"label\":\"A\",\"type\":\"foundation.isothermal_liquid.isothermal_liquid\"}],\"Top\":[]}"
  ReleaseCommand : PMIOPort  Side=Left
  PressurizeCommand : PMIOPort  Port=2  Side=Left
  ToBrake : PMIOPort  Port=3  Side=Right
  FromPrimaryCylinder : PMIOPort  Port=4  Side=Left
  connections:
  2-Position Valve Actuator2/LConn1 -- ReleaseCommand/RConn1
  PS Gain/LConn1 -- 2-Position Valve Actuator2/RConn1
  2-Position Valve Actuator1/LConn1 -- PressurizeCommand/RConn1
  PS Gain1/LConn1 -- 2-Position Valve Actuator1/RConn1
  Hydraulic Constant Pressure Source1/LConn1 -- Hydraulic Reference/LConn1
  Hydraulic Flow Rate Source1/LConn1 -- Hydraulic Reference1/LConn1
  Hydraulic Flow Rate Sensor1/RConn3 -- Hydraulic Flow Rate Source1/LConn2
  Orifice Release/LConn2 -- PS Gain/RConn1
  PS Gain1/RConn1 -- Orifice Apply/LConn2
  CV1/LConn1 -- Spring-Loaded Accumulator/RConn1 -- Orifice Release/LConn1
  ToBrake/RConn1 -- Orifice Release/RConn1 -- Orifice Apply/RConn1
  FromPrimaryCylinder/RConn1 -- Orifice Apply/LConn1 -- Hydraulic Flow Rate Source1/RConn1
  Hydraulic Flow Rate Sensor1/RConn1 -- Hydraulic Constant Pressure Source1/RConn1
  CV1/RConn1 -- Hydraulic Flow Rate Sensor1/LConn1

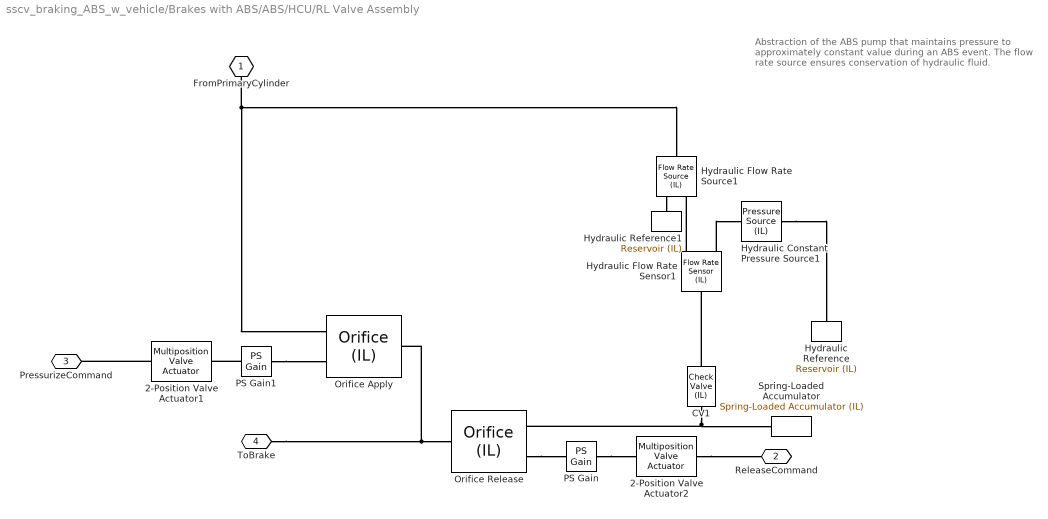
== system sscv_braking_ABS_w_vehicle/Brakes with ABS/ABS/HCU/RL Valve Assembly ==
  note: Abstraction of the ABS pump
      | that maintains pressure to
      | approximately constant value
      | during an ABS event. The
      | flow rate source ensures
      | conservation of hydraulic fluid.
  2-Position Valve Actuator1 : SimscapeFluids_lib/Valve Actuators/Multiposition Valve Actuator  positions=fluids.valve_actuators.enum.actuator_num_positions.two  stroke=HCU.PushPinS m  t_on=HCU.SwitchOnT s  t_off=HCU.SwitchOffT s  act_signal=HCU.NomSigV  init_position_2=0  init_position_3=fluids.valve_actuators.enum.actuator_three_pos_ic.neutral  act_orientation=1  local_time_specify=off  local_time_priority=None  local_time=0 s  local_time_nominal_specify=off  local_time_nominal_value=1  local_time_nominal_unit=s
      settings: InternalSimscapePortConfiguration="{\"Bottom\":[],\"Left\":[{\"id\":\"A\",\"label\":\"A\",\"type\":\"input\"}],\"Right\":[{\"id\":\"S\",\"label\":\"S\",\"type\":\"output\"}],\"Top\":[]}"
  2-Position Valve Actuator2 : SimscapeFluids_lib/Valve Actuators/Multiposition Valve Actuator  positions=fluids.valve_actuators.enum.actuator_num_positions.two  stroke=HCU.PushPinS m  t_on=HCU.SwitchOnT s  t_off=HCU.SwitchOffT s  act_signal=HCU.NomSigV  init_position_2=0  init_position_3=fluids.valve_actuators.enum.actuator_three_pos_ic.neutral  act_orientation=1  local_time_specify=off  local_time_priority=None  local_time=0 s  local_time_nominal_specify=off  local_time_nominal_value=1  local_time_nominal_unit=s
      settings: InternalSimscapePortConfiguration="{\"Bottom\":[],\"Left\":[{\"id\":\"A\",\"label\":\"A\",\"type\":\"input\"}],\"Right\":[{\"id\":\"S\",\"label\":\"S\",\"type\":\"output\"}],\"Top\":[]}"
  CV1 : SimscapeFluids_lib/Isothermal Liquid/Valves & Orifices/Directional Control Valves/Check Valve (IL)  opening_spec=fluids.isothermal_liquid.valves_orifices.enum.PressureOpeningSpec.Linear  pressure_control_spec=fluids.isothermal_liquid.valves_orifices.enum.pressure_control_spec.dp  p_crack_differential=HCU.cv1CrackP Pa  p_crack_gauge=0.1 MPa  press_max_differential=HCU.cv1MaxOpP Pa  press_max_gauge=0.2 MPa  area_max=HCU.cv1Amax m^2  area_leak=1e-8 m^2  p_diff_TLU=[0.01 : 0.01 : 0.1] MPa  valve_area_TLU=[1e-10, 1e-05, 2e-05, 3e-05, 4e-05, 5e-05, 6e-05, 7.5e-05, 8.5e-05, .0001] m^2  vol_flow_TLU=[.000358, .045, .11, .191, .284, .39, .505, .63, .764, .905] .* 1e-3 m^3/s  area=inf m^2  Cd=0.7  Re_c=150  smoothing_factor=0  pressure_recovery=simscape.enum.onoff.off  opening_dynamics=0  tau=0.1 s  enable_faults=simscape.enum.onoff.off  fault_action=fluids.enum.FaultOpening.Closed
      settings: InternalSimscapePortConfiguration="{\"Bottom\":[],\"Left\":[{\"id\":\"A\",\"label\":\"A\",\"type\":\"foundation.isothermal_liquid.isothermal_liquid\"}],\"Right\":[{\"id\":\"B\",\"label\":\"B\",\"type\":\"foundation.isothermal_liquid.isothermal_liquid\"}],\"Top\":[]}"
  Hydraulic Constant Pressure Source1 : fl_lib/Isothermal Liquid/Sources/Pressure Source (IL)  source_type=1  pressure_differential=1 atm
      settings: InternalSimscapePortConfiguration="{\"Bottom\":[],\"Left\":[{\"id\":\"A\",\"label\":\"A\",\"type\":\"foundation.isothermal_liquid.isothermal_liquid\"}],\"Right\":[{\"id\":\"B\",\"label\":\"B\",\"type\":\"foundation.isothermal_liquid.isothermal_liquid\"}],\"Top\":[]}"
  Hydraulic Flow Rate Sensor1 : fl_lib/Isothermal Liquid/Sensors/Flow Rate Sensor (IL)  sensor_type=3
      settings: InternalSimscapePortConfiguration="{\"Bottom\":[],\"Left\":[{\"id\":\"A\",\"label\":\"A\",\"type\":\"foundation.isothermal_liquid.isothermal_liquid\"}],\"Right\":[{\"id\":\"B\",\"label\":\"B\",\"type\":\"foundation.isothermal_liquid.isothermal_liquid\"},{\"id\":\"M\",\"label\":\"M\",\"type\":\"output\"},{\"id\":\"V\",\"label\":\"V\",\"type\":\"output\"}],\"Top\":[]}"
  Hydraulic Flow Rate Source1 : fl_lib/Isothermal Liquid/Sources/Flow Rate Source (IL)  source_type=foundation.enum.constant_controlled.controlled  flow_type=2  mass_flow=0 kg/s  volumetric_flow=0 m^3/s
      settings: InternalSimscapePortConfiguration="{\"Bottom\":[],\"Left\":[{\"id\":\"A\",\"label\":\"A\",\"type\":\"foundation.isothermal_liquid.isothermal_liquid\"},{\"id\":\"V\",\"label\":\"V\",\"type\":\"input\"}],\"Right\":[{\"id\":\"B\",\"label\":\"B\",\"type\":\"foundation.isothermal_liquid.isothermal_liquid\"}],\"Top\":[]}"
  Hydraulic Reference : fl_lib/Isothermal Liquid/Elements/Reservoir (IL)  reservoir_type=foundation.enum.constant_controlled.constant  pressure_spec=foundation.enum.pressure_spec.atmospheric  reservoir_pressure=0.101325 MPa
  Hydraulic Reference1 : fl_lib/Isothermal Liquid/Elements/Reservoir (IL)  reservoir_type=foundation.enum.constant_controlled.constant  pressure_spec=foundation.enum.pressure_spec.atmospheric  reservoir_pressure=0.101325 MPa
  Orifice Apply : SimscapeFluids_lib/Isothermal Liquid/Valves & Orifices/Orifices/Orifice (IL)  orifice_type=foundation.enum.constant_variable.variable  constant_orifice_spec=fluids.isothermal_liquid.valves_orifices.orifices.enum.constant_orifice_spec.area  variable_orifice_spec=1  orifice_area_constant=1e-3 m^2  p_diff_TLU_constant=[-4, -3, -2, -1, -.5, 0, .5, 1, 2, 3, 4] MPa  vol_flow_TLU_constant=[-2.44, -2.12, -1.68, -1.22, -.84, 0, .85, 1.21, 1.7, 2.09, 2.41] .* 1e-3 m^3/s  S_min=HCU.valve_x0 m  del_S=HCU.valve_maxO m  open_orientation=1  area_max=HCU.valve_maxA m^2  area_leak=HCU.valve_leak m^2  S_TLU=[-.002, 0, .002, .005, .015] - (HCU.valve_x0) m  orifice_area_TLU=[1e-09, 2.0352e-07, 4.0736e-05, .00011438, .00034356] m^2  area=inf m^2  Cd=0.7  Re_c=150  smoothing_factor=0  pressure_recovery=simscape.enum.onoff.off  S_vol_flow_TLU=[-.002, 0, .002, .005, .015] - (HCU.valve_x0) m  p_diff_TLU=[-10000000, -5000000, -2000000, 2000000, 5000000, 10000000] Pa  vol_flow_TLU=[-1e-07, -7.0711e-08, -4.4721e-08, 4.4721e-08, 7.0711e-08, 1e-07; -2.0352e-05, -1.4391e-05, -9.1017e-06, 9.1017e-06, 1.4391e-05, 2.0352e-05; -.0040736, -.0028805, -.0018218, .0018218, .0028805, .0040736; -.011438, -.0080879, -.0051152, .0051152, .0080879, .011438; -.034356, -.024293, -.015364, .015364, .024293, .034356] m^3/s  enable_faults=simscape.enum.onoff.off  fault_action=fluids.enum.FaultOpening.Closed
      settings: InternalSimscapePortConfiguration="{\"Bottom\":[],\"Left\":[{\"id\":\"A\",\"label\":\"A\",\"type\":\"foundation.isothermal_liquid.isothermal_liquid\"},{\"id\":\"S\",\"label\":\"S\",\"type\":\"input\"}],\"Right\":[{\"id\":\"B\",\"label\":\"B\",\"type\":\"foundation.isothermal_liquid.isothermal_liquid\"}],\"Top\":[]}"
  Orifice Release : SimscapeFluids_lib/Isothermal Liquid/Valves & Orifices/Orifices/Orifice (IL)  orifice_type=foundation.enum.constant_variable.variable  constant_orifice_spec=fluids.isothermal_liquid.valves_orifices.orifices.enum.constant_orifice_spec.area  variable_orifice_spec=1  orifice_area_constant=1e-3 m^2  p_diff_TLU_constant=[-4, -3, -2, -1, -.5, 0, .5, 1, 2, 3, 4] MPa  vol_flow_TLU_constant=[-2.44, -2.12, -1.68, -1.22, -.84, 0, .85, 1.21, 1.7, 2.09, 2.41] .* 1e-3 m^3/s  S_min=HCU.valve_x0 m  del_S=HCU.valve_maxO m  open_orientation=1  area_max=HCU.valve_maxA m^2  area_leak=HCU.valve_leak m^2  S_TLU=[-.002, 0, .002, .005, .015] - (HCU.valve_x0) m  orifice_area_TLU=[1e-09, 2.0352e-07, 4.0736e-05, .00011438, .00034356] m^2  area=inf m^2  Cd=0.7  Re_c=150  smoothing_factor=0  pressure_recovery=simscape.enum.onoff.off  S_vol_flow_TLU=[-.002, 0, .002, .005, .015] - (HCU.valve_x0) m  p_diff_TLU=[-10000000, -5000000, -2000000, 2000000, 5000000, 10000000] Pa  vol_flow_TLU=[-1e-07, -7.0711e-08, -4.4721e-08, 4.4721e-08, 7.0711e-08, 1e-07; -2.0352e-05, -1.4391e-05, -9.1017e-06, 9.1017e-06, 1.4391e-05, 2.0352e-05; -.0040736, -.0028805, -.0018218, .0018218, .0028805, .0040736; -.011438, -.0080879, -.0051152, .0051152, .0080879, .011438; -.034356, -.024293, -.015364, .015364, .024293, .034356] m^3/s  enable_faults=simscape.enum.onoff.off  fault_action=fluids.enum.FaultOpening.Closed
      settings: InternalSimscapePortConfiguration="{\"Bottom\":[],\"Left\":[{\"id\":\"A\",\"label\":\"A\",\"type\":\"foundation.isothermal_liquid.isothermal_liquid\"},{\"id\":\"S\",\"label\":\"S\",\"type\":\"input\"}],\"Right\":[{\"id\":\"B\",\"label\":\"B\",\"type\":\"foundation.isothermal_liquid.isothermal_liquid\"}],\"Top\":[]}"
  PS Gain : fl_lib/Physical Signals/Functions/PS Gain  gain=HCU.valve_maxO
  PS Gain1 : fl_lib/Physical Signals/Functions/PS Gain  gain=HCU.valve_maxO
  Spring-Loaded Accumulator : SimscapeFluids_lib/Isothermal Liquid/Tanks & Accumulators/Spring-Loaded Accumulator (IL)  capacity=HCU.FluidChamC cm^3  p_preload="HCU.PrelP  bar"  p_max="HCU.FullCapP  bar"  stiff_coeff=HCU.hss Pa/m^3  dynamic_compressibility=simscape.enum.onoff.off  liquid_volume_specify=on  liquid_volume_priority=High  liquid_volume=0 m^3  liquid_volume_nominal_specify=off  liquid_volume_nominal_value=1  liquid_volume_nominal_unit=m^3  liquid_mass_specify=off  liquid_mass_priority=None  liquid_mass=5 kg  liquid_mass_nominal_specify=off  liquid_mass_nominal_value=1  liquid_mass_nominal_unit=kg  p_I_specify=on  p_I_priority=None  p_I=1.01325e5 Pa  p_I_nominal_specify=off  p_I_nominal_value=1  p_I_nominal_unit=Pa
      settings: InternalSimscapePortConfiguration="{\"Bottom\":[],\"Left\":[],\"Right\":[{\"id\":\"A\",\"label\":\"A\",\"type\":\"foundation.isothermal_liquid.isothermal_liquid\"}],\"Top\":[]}"
  FromPrimaryCylinder : PMIOPort  Side=Left
  ReleaseCommand : PMIOPort  Port=2  Side=Left
  PressurizeCommand : PMIOPort  Port=3  Side=Left
  ToBrake : PMIOPort  Port=4  Side=Right
  connections:
  2-Position Valve Actuator2/LConn1 -- ReleaseCommand/RConn1
  PS Gain/LConn1 -- 2-Position Valve Actuator2/RConn1
  2-Position Valve Actuator1/LConn1 -- PressurizeCommand/RConn1
  PS Gain1/LConn1 -- 2-Position Valve Actuator1/RConn1
  Hydraulic Constant Pressure Source1/LConn1 -- Hydraulic Reference/LConn1
  Hydraulic Flow Rate Source1/LConn1 -- Hydraulic Reference1/LConn1
  Hydraulic Flow Rate Sensor1/RConn3 -- Hydraulic Flow Rate Source1/LConn2
  Orifice Release/LConn2 -- PS Gain/RConn1
  PS Gain1/RConn1 -- Orifice Apply/LConn2
  CV1/LConn1 -- Spring-Loaded Accumulator/RConn1 -- Orifice Release/LConn1
  ToBrake/RConn1 -- Orifice Release/RConn1 -- Orifice Apply/RConn1
  FromPrimaryCylinder/RConn1 -- Orifice Apply/LConn1 -- Hydraulic Flow Rate Source1/RConn1
  Hydraulic Flow Rate Sensor1/RConn1 -- Hydraulic Constant Pressure Source1/RConn1
  CV1/RConn1 -- Hydraulic Flow Rate Sensor1/LConn1
